simulink model "test_model_1"  (R2020b)
settings: Solver=VariableStepAuto  StartTime=0.0  StopTime=inf  RelTol=1e-3
values from neighbouring files (symbols this model uses):
  AUV = struct    [Parameters_2.m]
  HydroDyn = struct    [Parameters_2.m]
  kc = 57.2958    [Calculations.m]    (also in Parameters_2.m)
  Vfwd = Vfwd(2)    [Parameters_2.m]
  Vz = 0    [Parameters_2.m]
  Z_delay = 0.01    [Parameters_2.m]
libraries: simulink x3, slrealtimeutilitieslib x2, slrealtimeiplib x2, simulink_extras x1, sldrtlib x1
settings Model: Creator=117-11  LastModifiedBy=corsair
settings DataIOCC: ReturnWorkspaceOutputs=off
settings DebuggingCC: ArithmeticOperatorsInVariantConditions=warning
settings SFSimCC: CustomCodeUndefinedFunction=UseInterfaceOnly

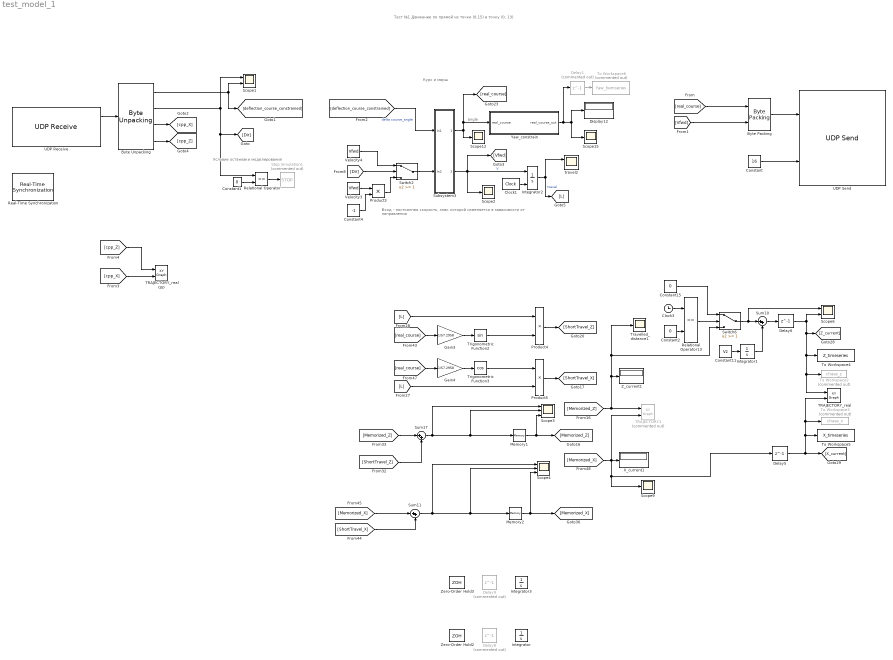
== system test_model_1 ==
  note: Тест №1
      | Движение по прямой из точки (0,15) в точку (0, 13)
  note: Вход - постоянная скорость, знак которой изменяется в зависимости от направления
  note: angle
  note: Курс и марш
  note: Условие остановки моделирования
  "Byte Packing " : slrealtimeutilitieslib/Byte Packing  MaskPackedDataType=uint8  MaskUnpackedDataTypes={'double', 'double'}  MaskAlignment=1
  "Byte Unpacking " : slrealtimeutilitieslib/Byte Unpacking  MaskUnpackedDataTypes={'double', 'double', 'double', 'double'}  MaskUnpackedDataSizes={[1], [1], [1], [1]}  MaskAlignment=1
      settings: SourceProductBaseCode=XP
  Clock1 : simulink_extras/Flip Flops/Clock  period=Z_delay
  Clock3 : Clock
  Constant : Constant  Value=16
  Constant1 : Constant  Value=0
  Constant11 : Constant  Value=Vz
  Constant15 : Constant  Value=0
  Constant2 : Constant  Value=0
  Constant4 : Constant  Value=-1
  Delay1 : Delay  Commented=on  DelayLength=1  InitialCondition=180  SampleTime=Z_delay
  Delay5 : Delay  DelayLength=1  InitialCondition=15  SampleTime=0.1
  Delay6 : Delay  DelayLength=1  SampleTime=0.1
  Delay8 : Delay  Commented=on  DelayLength=1  InitialCondition=15
  Delay9 : Delay  Commented=on  DelayLength=1
  Display12 : Display
  Gain3 : Gain  Gain=1/57.2958
  Gain4 : Gain  Gain=1/57.2958
  Integrator : Integrator  InitialCondition=15
  Integrator1 : Integrator
  Integrator2 : Integrator  ExternalReset=rising
  Integrator3 : Integrator
  Memory1 : Memory  InheritSampleTime=on  LinearizeMemory=on
  Memory2 : Memory  InitialCondition=15  InheritSampleTime=on  LinearizeMemory=on
  Product3 : Product
  Product4 : Product
  Product5 : Product
  Real-Time Synchronization : sldrtlib/Real-Time Synchronization  SampleTime=0.001  MaxMissedTicks=10  ShowMissedTicks=off  YieldWhenWaiting=off
  Relational Operator : RelationalOperator  Operator===  OutDataTypeStr=boolean  RndMeth=Simplest
  Relational Operator13 : RelationalOperator  Operator===  OutDataTypeStr=boolean  RndMeth=Simplest
  Scope1 : Scope  NumInputPorts=2
  Scope{2,9,12,15} (4 alike) : Scope
  Scope3 : Scope  NumInputPorts=3
  Scope4 : Scope  NumInputPorts=3
  Scope6 : Scope  NumInputPorts=2
  Stop Simulation1 : Stop  Commented=on
  Subsystem3 : Subsystem
  Sum10 : Sum  Inputs=|++
  Sum11 : Sum  Inputs=|++
  Sum17 : Sum  Inputs=|++
  Switch2 : Switch  Threshold=1
  Switch6 : Switch  Threshold=1
  TRAJECTORY1 : simulink/Sinks/XY Graph  Commented=on  xmin=-15  xmax=15  ymin=-15  ymax=15  st=-1
  TRAJECTORY_real : simulink/Sinks/XY Graph  xmin=-15  xmax=15  ymin=-15  ymax=15  st=-1
  TRAJECTORY_real cpp : simulink/Sinks/XY Graph  xmin=-15  xmax=15  ymin=-15  ymax=15  st=Z_delay
  To Workspace2 : ToWorkspace  Commented=on  VariableName=chase_z  SampleTime=-1
  To Workspace3 : ToWorkspace  Commented=on  VariableName=chase_x  SampleTime=-1
  To Workspace4 : ToWorkspace  VariableName=Z_timeseries  SaveFormat=Timeseries  SampleTime=-1
  To Workspace5 : ToWorkspace  VariableName=X_timeseries  SaveFormat=Timeseries  SampleTime=-1
  To Workspace6 : ToWorkspace  Commented=on  VariableName=Yaw_tiemseries  SaveFormat=Timeseries  SampleTime=-1
  Travelled_distance1 : Scope
  Trigonometric Function2 : Trigonometry
  Trigonometric Function3 : Trigonometry  Operator=cos
  UDP Receive : slrealtimeiplib/UDP Receive  useHostTargetConn=on  ipAddress=10.10.10.15  localPort=13042  rcvWidth=32  rcvFmAny=on  fmAddress=0.0.0.0  rcvMulticast=off  multicastAddress={}  sampleTime=-1
      settings: SourceProductBaseCode=XP
  UDP Send : slrealtimeiplib/UDP Send  useHostTargetConn=on  ipAddress=10.10.10.15  localPort=13043  toAddress=127.0.0.1  toPort=13044  sampleTime=0.001
      settings: SourceProductBaseCode=XP
  Velocity3 : Constant  Value=Vfwd
  Velocity4 : Constant  Value=Vfwd
  X_current1 : Display
  Yaw_constrain : MATLAB Function  TreatAsAtomicUnit=on
  Z_current1 : Display
  Zero-Order Hold2 : ZeroOrderHold  SampleTime=0.033
  Zero-Order Hold3 : ZeroOrderHold  SampleTime=0.033
  travel2 : Scope  NumInputPorts=2
  wires:
  "Byte Unpacking "/1 -> [deflection_course_constrained], Scope1/2
  UDP Receive/1 -> "Byte Unpacking "/1
  [real_course] -> "Byte Packing "/1
  Constant/1 -> UDP Send/2
  "Byte Packing "/1 -> UDP Send/1
  Velocity4/1 -> Switch2/1
  Velocity3/1 -> Product3/1
  Switch2/1 -> Subsystem3/2(In2)
  Product3/1 -> Switch2/3
  Constant4/1 -> Product3/2
  [Dir] -> Switch2/2
  [deflection_course_constrained] -> Subsystem3/1(In1)  "delta course_angle"
  Delay1/1 -> To Workspace6/1
  Subsystem3/1(Out1) -> [real_course], Yaw_constrain/1(real_course), Scope12/1
  Yaw_constrain/1(real_course_out) -> Delay1/1, Scope15/1, Display12/1
  "Byte Unpacking "/2 -> Relational Operator/1, [Dir], Scope1/1
  [Vfwd] -> "Byte Packing "/2
  [Memorized_Z] -> Switch6/3, Travelled_distance1/1, Z_current1/1, TRAJECTORY1/1
  [ShortTravel_X] -> Sum11/2
  Gain3/1 -> Trigonometric Function2/1
  Integrator1/1 -> Sum10/2
  Constant15/1 -> Switch6/1
  Trigonometric Function2/1 -> Product4/2
  Clock3/1 -> Relational Operator13/1
  Trigonometric Function3/1 -> Product5/1
  Memory2/1 -> Scope4/3, [Memorized_X]
  Sum11/1 -> Memory2/1, Scope4/2, Scope4/1
  [real_course] -> Gain4/1
  Gain4/1 -> Trigonometric Function3/1
  Sum17/1 -> Memory1/1, Scope3/2, Scope3/1
  [Memorized_X] -> Scope9/1, Delay5/1, TRAJECTORY1/2, X_current1/1
  [Memorized_X] -> Sum11/1
  Delay6/1 -> To Workspace4/1, TRAJECTORY_real/1, To Workspace2/1, [Z_current], Scope6/2
  Constant2/1 -> Relational Operator13/2
  Memory1/1 -> Scope3/3, [Memorized_Z]
  Product4/1 -> [ShortTravel_Z]
  Delay5/1 -> [X_current], To Workspace5/1, TRAJECTORY_real/2, To Workspace3/1
  Constant11/1 -> Integrator1/1
  [L] -> Product5/2
  Relational Operator13/1 -> Switch6/2
  [L] -> Product4/1
  [Memorized_Z] -> Sum17/1
  Switch6/1 -> Scope6/1, Sum10/1
  Sum10/1 -> Delay6/1
  [ShortTravel_Z] -> Sum17/2
  [real_course] -> Gain3/1
  Product5/1 -> [ShortTravel_X]
  Integrator2/1 -> travel2/1, [L]  "travel"
  Clock1/1 -> Integrator2/2
  Subsystem3/2(Out2) -> [Vfwd], Integrator2/1, Scope2/1  "V"
  Relational Operator/1 -> Stop Simulation1/1
  Constant1/1 -> Relational Operator/2
  "Byte Unpacking "/3 -> [cpp_X]
  "Byte Unpacking "/4 -> [cpp_Z]
  [cpp_X] -> TRAJECTORY_real cpp/2
  [cpp_Z] -> TRAJECTORY_real cpp/1

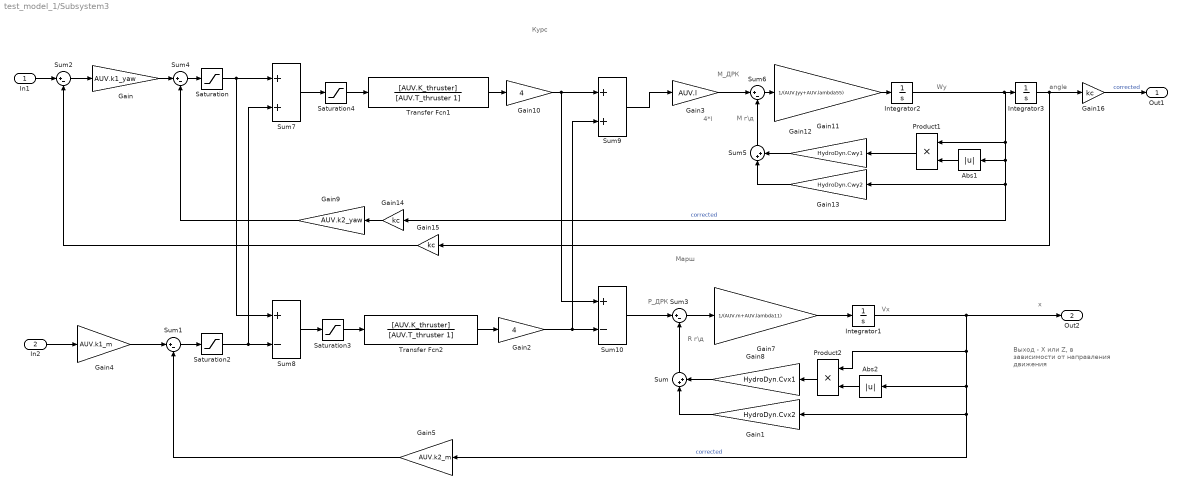
== system test_model_1/Subsystem3 ==
  note: Курс
  note: Wy
  note: M_ДРК
  note: 4*l
  note: angle
  note: M г\д
  note: Марш
  note: x
  note: R г\д
  note: P_ДРК
  note: Vx
  note: Выход - X или Z, в зависимости от направления движения
  In1 : Inport
  In2 : Inport  Port=2
  Abs1 : Abs
  Abs2 : Abs
  Gain : Gain  Gain=AUV.k1_yaw
  Gain1 : Gain  Gain=HydroDyn.Cvx2
  Gain10 : Gain  Gain=4
  Gain11 : Gain  Gain=1/(AUV.Jyy+AUV.lambda55)
  Gain12 : Gain  Gain=HydroDyn.Cwy1
  Gain13 : Gain  Gain=HydroDyn.Cwy2
  Gain14 : Gain  Gain=kc
  Gain15 : Gain  Gain=kc
  Gain16 : Gain  Gain=kc
  Gain2 : Gain  Gain=4
  Gain3 : Gain  Gain=AUV.l
  Gain4 : Gain  Gain=AUV.k1_m
  Gain5 : Gain  Gain=AUV.k2_m
  Gain7 : Gain  Gain=1/(AUV.m+AUV.lambda11)
  Gain8 : Gain  Gain=HydroDyn.Cvx1
  Gain9 : Gain  Gain=AUV.k2_yaw
  Integrator1 : Integrator  InitialCondition=0.7
  Integrator2 : Integrator
  Integrator3 : Integrator  InitialCondition=3.1416
  Product1 : Product
  Product2 : Product
  Saturation : Saturate  UpperLimit=24  LowerLimit=-24
  Saturation2 : Saturate  UpperLimit=24  LowerLimit=-24
  Saturation3 : Saturate  UpperLimit=12  LowerLimit=-12
  Saturation4 : Saturate  UpperLimit=12  LowerLimit=-12
  Sum : Sum  Inputs=|++
  Sum{1..4,6} (5 alike) : Sum  Inputs=|+-
  Sum10 : Sum  Inputs=+-
  Sum5 : Sum  Inputs=|++
  Sum7 : Sum
  Sum8 : Sum  Inputs=+-
  Sum9 : Sum
  Transfer Fcn1 : TransferFcn  Numerator=[AUV.K_thruster]  Denominator=[AUV.T_thruster 1]
  Transfer Fcn2 : TransferFcn  Numerator=[AUV.K_thruster]  Denominator=[AUV.T_thruster 1]
  Out1 : Outport  VectorParamsAs1DForOutWhenUnconnected=off
  Out2 : Outport  Port=2  VectorParamsAs1DForOutWhenUnconnected=off
  wires:
  Gain12/1 -> Sum5/2
  Product1/1 -> Gain12/1
  Gain11/1 -> Integrator2/1
  Gain9/1 -> Sum4/2
  Gain/1 -> Sum4/1
  Transfer Fcn1/1 -> Gain10/1
  Sum6/1 -> Gain11/1
  Gain14/1 -> Gain9/1
  Gain15/1 -> Sum2/2
  Gain13/1 -> Sum5/1
  Abs1/1 -> Product1/2
  Sum5/1 -> Sum6/2
  Integrator2/1 -> Integrator3/1, Abs1/1, Gain14/1, Gain13/1, Product1/1  "corrected"
  Sum2/1 -> Gain/1
  Integrator3/1 -> Gain16/1, Gain15/1
  In1/1 -> Sum2/1
  Gain16/1 -> Out1/1  "corrected"
  Sum4/1 -> Saturation/1
  Integrator1/1 -> Gain5/1, Gain1/1, Abs2/1, Product2/1, Out2/1  "corrected"
  Sum1/1 -> Saturation2/1
  Gain7/1 -> Integrator1/1
  Sum3/1 -> Gain7/1
  Abs2/1 -> Product2/2
  Gain1/1 -> Sum/1
  Gain4/1 -> Sum1/1
  Gain8/1 -> Sum/2
  Transfer Fcn2/1 -> Gain2/1
  Sum/1 -> Sum3/2
  Gain5/1 -> Sum1/2
  In2/1 -> Gain4/1
  Product2/1 -> Gain8/1
  Saturation/1 -> Sum8/1, Sum7/1
  Sum7/1 -> Saturation4/1
  Saturation4/1 -> Transfer Fcn1/1
  Saturation2/1 -> Sum7/2, Sum8/2
  Sum8/1 -> Saturation3/1
  Saturation3/1 -> Transfer Fcn2/1
  Gain3/1 -> Sum6/1
  Gain10/1 -> Sum9/1, Sum10/1
  Sum9/1 -> Gain3/1
  Gain2/1 -> Sum9/2, Sum10/2
  Sum10/1 -> Sum3/1

== matlab function test_model_1/Yaw_constrain ==
  data: real_course input; real_course_out output
function real_course_out   = fcn(real_course)

    % Приводим к стандарту
    if real_course < 0
        real_course_out = 360 - abs(real_course);
    elseif real_course >= 360
        real_course_out = real_course - 360;
    else    
        real_course_out = real_course;
    end

end
